simulink model "Model"  (R2025a)
settings: Solver=VariableStepAuto  StartTime=0.0  StopTime=10.0  RelTol=1e-3
settings Model: Creator=thinkpad  LastModifiedBy=thinkpad

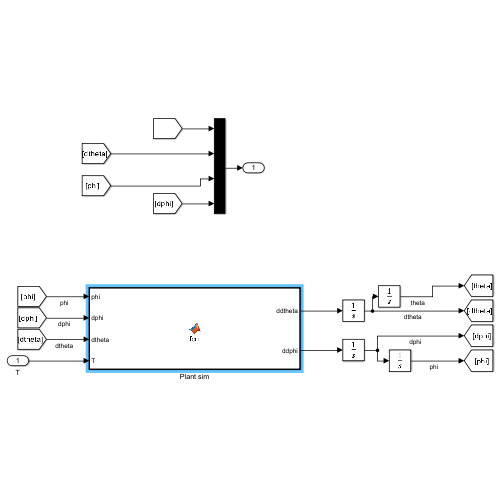
[thumbnail: Simulink's stored preview of the top-level diagram]
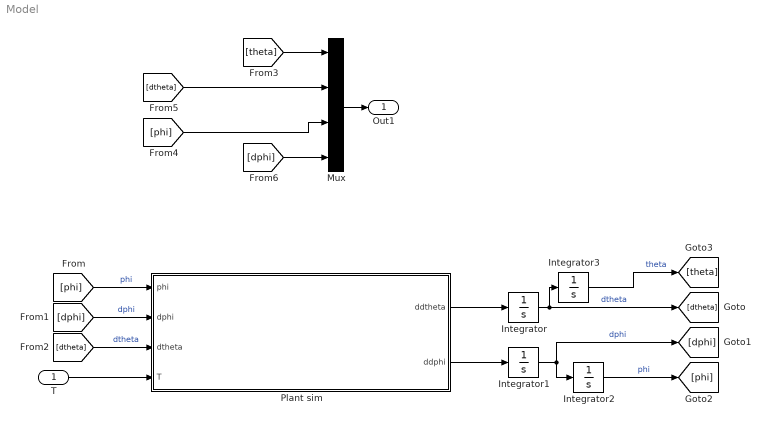
== system Model ==
  T : Inport
  Integrator : Integrator
  Integrator1 : Integrator
  Integrator2 : Integrator
  Integrator3 : Integrator  InitialCondition=pi
  Mux : Mux
  Plant sim : MATLAB Function  TreatAsAtomicUnit=on
  Out1 : Outport
  wires:
  Plant sim/2(ddphi) -> Integrator1/1
  Integrator1/1 -> [dphi], Integrator2/1  "dphi"
  Plant sim/1(ddtheta) -> Integrator/1
  Integrator/1 -> Integrator3/1, [dtheta]  "dtheta"
  Integrator2/1 -> [phi]  "phi"
  [dtheta] -> Plant sim/3(dtheta)  "dtheta"
  [dphi] -> Plant sim/2(dphi)  "dphi"
  [phi] -> Plant sim/1(phi)  "phi"
  Integrator3/1 -> [theta]  "theta"
  [theta] -> Mux/1
  [phi] -> Mux/3
  [dtheta] -> Mux/2
  [dphi] -> Mux/4
  Mux/1 -> Out1/1
  T/1 -> Plant sim/4(T)

== matlab function Model/Plant sim ==
  data: phi input; ddtheta output; dphi input; dtheta input; T input; ddphi output
function [ddtheta, ddphi] = fcn(phi, dphi, dtheta, T)

R = 0.3700
l = 0.2698
r = 0; %reduced into J1_bar
M = 0; %reduced into J1_bar
g = 9.81;
c1 = 1; %friction of base
c2 = 0; %friction of pivot

% J =  0.1530 % J1_bar J - inertia of the table
J =  0.1314 
Ixx = 0
Iyy = 5.5625e-05 %Jy 
Izz = 0.0131%Jz_bar%  I - inertia of the pendulum
% Izz = 0.0132
m =     0.1580
T = T;


ddphi = (0.5000*Iyy*dtheta^2*sin(2*phi) - g*l*m*sin(phi) + 0.5000*dtheta^2*l^2*m*sin(2*phi) - (R*l*m*cos(phi)*(R*m*sin(phi)*dphi^2*l + dtheta*m*sin(2*phi)*dphi*l^2 + Iyy*dtheta*sin(2*phi)*dphi - T + c1*dtheta))/(m*R^2 - m*l^2*cos(phi)^2 + m*l^2 - Iyy*cos(phi)^2 + Iyy + J))/(Izz + l^2*m - (R^2*l^2*m^2*cos(phi)^2)/(m*R^2 - m*l^2*cos(phi)^2 + m*l^2 - Iyy*cos(phi)^2 + Iyy + J))

% ddphi = -(0.5000*Iyy*dtheta^2*sin(2*phi) - g*l*m*sin(phi) + 0.5000*dtheta^2*l^2*m*sin(2*phi) + (R*l*m*cos(phi)*(- R*m*sin(phi)*dphi^2*l + dtheta*m*sin(2*phi)*dphi*l^2 + Iyy*dtheta*sin(2*phi)*dphi - T + c1*dtheta))/(m*R^2 - m*l^2*cos(phi)^2 + m*l^2 - Iyy*cos(phi)^2 + Iyy + J))/(Izz + l^2*m - (R^2*l^2*m^2*cos(phi)^2)/(m*R^2 - m*l^2*cos(phi)^2 + m*l^2 - Iyy*cos(phi)^2 + Iyy + J))

ddtheta =-(c1*dtheta - Izz*ddphi - T + 0.5000*Iyy*dtheta^2*sin(2*phi) - ddphi*l^2*m - g*l*m*sin(phi) + 0.5000*dtheta^2*l^2*m*sin(2*phi) + Iyy*dphi*dtheta*sin(2*phi) + R*dphi^2*l*m*sin(phi) + dphi*dtheta*l^2*m*sin(2*phi) - R*ddphi*l*m*cos(phi))/(m*R^2 + m*R*l*cos(phi) - m*l^2*cos(phi)^2 + m*l^2 - Iyy*cos(phi)^2 + Iyy + J);

% ddtheta =-(- R*m*sin(phi)*dphi^2*l + dtheta*m*sin(2*phi)*dphi*l^2 + Iyy*dtheta*sin(2*phi)*dphi + R*ddphi*m*cos(phi)*l - T + c1*dtheta)/(m*R^2 - m*l^2*cos(phi)^2 + m*l^2 - Iyy*cos(phi)^2 + Iyy + J);
% ddtheta =-(- R*m*sin(phi)*dphi^2*l + dtheta*m*sin(2*phi)*dphi*l^2 + Iyy*dtheta*sin(2*phi)*dphi + R*ddphi*m*cos(phi)*l - T + c1*dtheta)/(m*R^2 - m*l^2*cos(phi)^2 + m*l^2 - Iyy*cos(phi)^2 + Iyy + J)
% ddtheta = -(c1*dtheta - Izz*ddphi - T + 0.5000*Iyy*dtheta^2*sin(2*phi) - ddphi*l^2*m - g*l*m*sin(phi) + 0.5000*dtheta^2*l^2*m*sin(2*phi) + Iyy*dphi*dtheta*sin(2*phi) - R*dphi^2*l*m*sin(phi) + dphi*dtheta*l^2*m*sin(2*phi) + R*ddphi*l*m*cos(phi))/(m*R^2 - m*R*l*cos(phi) - m*l^2*cos(phi)^2 + m*l^2 - Iyy*cos(phi)^2 + Iyy + J)
